simulink model "testsystem"  (R2023b)
settings: Solver=VariableStepAuto  StartTime=0.0  StopTime=50  RelTol=1e-3
values from neighbouring files (symbols this model uses):
  frontTrackWidth = 1.4    [SetVehicleParameters.m]    (also in SetVehicleParameters2.m = 1; SetVehicleParameters4.m = 1; SetVehicleParameters5.m = 1; SetVehicleParameters6.m = 1)
  g = 9.8    [SetVehicleParameters.m]    (also in SetVehicleParameters2.m; SetVehicleParameters4.m; SetVehicleParameters5.m; SetVehicleParameters6.m)
  L = Lf + Lr    (= 3)    [SetVehicleParameters.m]    (also in SetVehicleParameters2.m = 2; SetVehicleParameters4.m = 2; SetVehicleParameters5.m = 2; SetVehicleParameters6.m = 2)
  Lr = 1.6    [SetVehicleParameters.m]    (also in SetVehicleParameters2.m = 0.5; SetVehicleParameters4.m = 0.5; SetVehicleParameters5.m = 0.5; SetVehicleParameters6.m = 0.5)
  mass = 2000    [SetVehicleParameters.m]    (also in SetVehicleParameters2.m = 420; SetVehicleParameters4.m = 420; SetVehicleParameters5.m = 420; SetVehicleParameters6.m = 420)
  rearTrackWidth = 1.4    [SetVehicleParameters.m]    (also in SetVehicleParameters2.m = 1; SetVehicleParameters4.m = 1; SetVehicleParameters5.m = 1; SetVehicleParameters6.m = 1)
libraries: vehdynlibsteering x1, slpidlib x1, vehdynlibviscommon x1, SignalEditorBlockLib x1, autolibshared x1
settings Model: Creator=denoc  LastModifiedBy=denoc

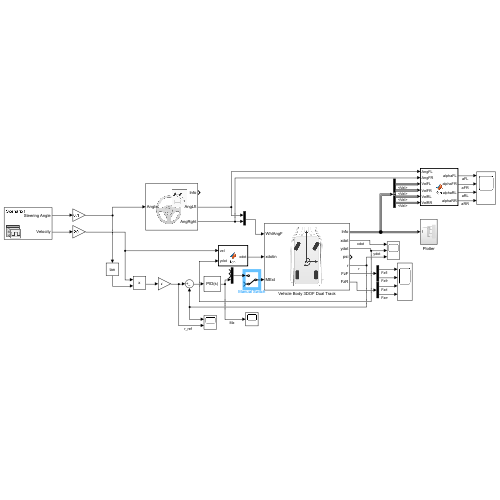
[thumbnail: Simulink's stored preview of the top-level diagram]
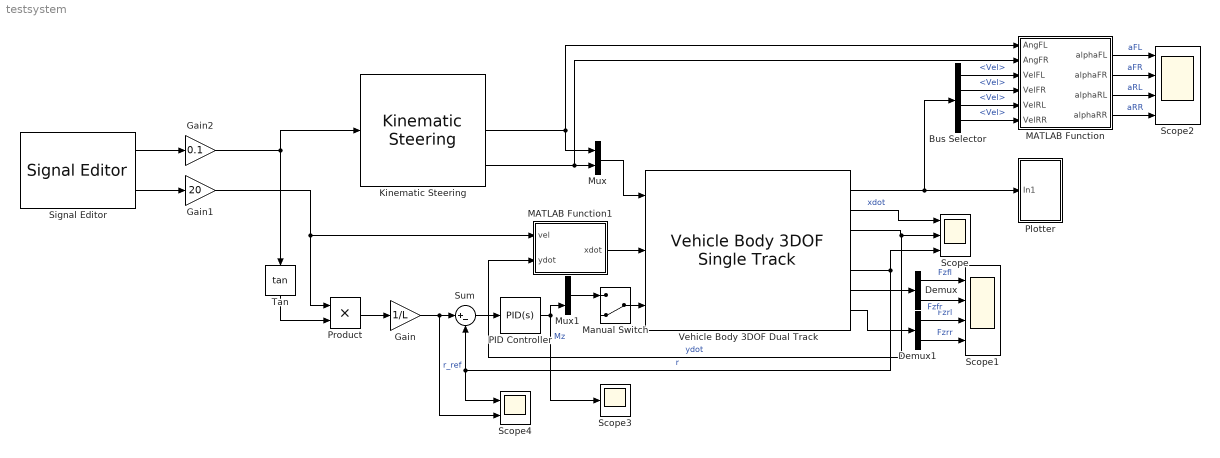
== system testsystem ==
  Bus Selector : BusSelector  OutputSignals=BdyFrm.FrntAxl.Lft.Vel,BdyFrm.FrntAxl.Rght.Vel,BdyFrm.RearAxl.Lft.Vel,BdyFrm.RearAxl.Rght.Vel
  Demux : Demux  Outputs=2
  Demux1 : Demux  Outputs=2
  Gain : Gain  Gain=1/L
  Gain1 : Gain  Gain=20
  Gain2 : Gain  Gain=0.1
  Kinematic Steering : vehdynlibsteering/Kinematic Steering  StrgType=Ackerman  StrgRatioType=Constant  Loc=Front  NrmlFctr=1  TrckWdth=frontTrackWidth  WhlBase=L  Db=0  StrgRng=1.25*pi  StrgAngBpts="[-6.2832   -5.0265   -3.7699   -2.5133   -1.2566         0    1.2566    2.5133    3.7699    5.0265    6.2832]"  StrgRatioTbl=|  StrgRatio=1  PctAckIn=off  PctAck=100  PctAckTbl=ones(1,11)*100  StrgArmLngth=0.1  RckCsLngth=0.5  TieRodLngth=0.248  D=0.2  PnnRadius=0.00085818  PnnRadiusTbl="[0.0055    0.0055    0.0056    0.0057    0.0058    0.0057    0.0057    0.0057    0.0056    0.0055    0.0055]"  RodLngth=0.1  ParaArmLngth=0.9  aMode=2
      | [13.5000   13.3750   13.2500   13.1250   13.0000   13.0000   13.0000   13.1250   13.2500   13.3750   13.5000
      | ]
  MATLAB Function : MATLAB Function  TreatAsAtomicUnit=on
  MATLAB Function1 : MATLAB Function  TreatAsAtomicUnit=on
  Manual Switch : ManualSwitch  CurrentSetting=0
  Mux : Mux  Inputs=2
  Mux1 : Mux  Inputs=3
  PID Controller : slpidlib/PID Controller  Controller=PID  Form=Parallel  TimeDomain=Continuous-time  UseExternalTs=off  SampleTime=-1  IntegratorMethod=Forward Euler  FilterMethod=Forward Euler  ControllerParametersSource=internal  P=50000  I=25000  UseKiTs=off  D=0  N=100  UseFilter=on  TunerSelectOption=Transfer Function Based (PID Tuner App)  InitialConditionSource=internal  InitialConditionForIntegrator=0  InitialConditionForFilter=0  DifferentiatorICPrevScaledInput=0  ExternalReset=none  TrackingMode=off  Kt=1  LimitOutput=off  SatLimitsSource=internal  UpperSaturationLimit=inf  LowerSaturationLimit=-inf  LinearizeAsGain=on  AntiWindupMode=none  Kb=1  LimitIntegrator=off  UpperIntegratorSaturationLimit=inf  LowerIntegratorSaturationLimit=-inf  POutMin=[]  POutMax=[]  IOutMin=[]  IOutMax=[]  DOutMin=[]  DOutMax=[]  NOutMin=[]  NOutMax=[]  SumOutMin=[]  SumOutMax=[]  SaturationOutMin=[]  SaturationOutMax=[]  PParamMin=[]  PParamMax=[]  IParamMin=[]  IParamMax=[]  DParamMin=[]  DParamMax=[]  NParamMin=[]  NParamMax=[]  KbParamMin=[]  KbParamMax=[]  KtParamMin=[]  KtParamMax=[]  KbOutMin=[]  KbOutMax=[]  KtOutMin=[]  KtOutMax=[]  IntegratorOutMin=[]  IntegratorOutMax=[]  FilterOutMin=[]  FilterOutMax=[]  SumI1OutMin=[]  SumI1OutMax=[]  SumI2OutMin=[]  SumI2OutMax=[]  SumI3OutMin=[]  SumI3OutMax=[]  SumI4OutMin=[]  SumI4OutMax=[]  SumDOutMin=[]  SumDOutMax=[]  DifferentiatorOutMin=[]  DifferentiatorOutMax=[]  FilterDiffOutCoefMin=[]  FilterDiffOutCoefMax=[]  ReciprocalOutMin=[]  ReciprocalOutMax=[]  SumDenOutMin=[]  SumDenOutMax=[]  SumNumOutMin=[]  SumNumOutMax=[]  DivideOutMin=[]  DivideOutMax=[]  UdiffTsProdOutMin=[]  UdiffTsProdOutMax=[]  NTsProdOutMin=[]  NTsProdOutMax=[]  UintegralTsProdOutMin=[]  UintegralTsProdOutMax=[]  UngainTsProdOutMin=[]  UngainTsProdOutMax=[]  ClampingZeroOutDataTypeStr=Inherit: Inherit via back propagation  ClampingZeroOutMin=[]  ClampingZeroOutMax=[]  FilterDenConstantOutDataTypeStr=Inherit: Inherit via back propagation  FilterDenConstantOutMin=[]  FilterDenConstantOutMax=[]  PCopyOutDataTypeStr=Inherit: Inherit via back propagation  PCopyOutMin=[]  PCopyOutMax=[]  NCopyOutDataTypeStr=Inherit: Inherit via back propagation  NCopyOutMin=[]  NCopyOutMax=[]  IntegratorContinuousStateAttributes=''  IntegratorStateMustResolveToSignalObject=off  IntegratorRTWStateStorageClass=Auto  FilterContinuousStateAttributes=''  FilterStateMustResolveToSignalObject=off  FilterRTWStateStorageClass=Auto  ParallelPVariant=InternalParameters  IdealPVariant=Disabled  IVariant=InternalParameters  DVariant=InternalParameters  IntegratorVariant=Continuous  SatVariant=Disabled  AWVariant=Passthrough  PCopyVariant=Disabled  TRVariant=Disabled  FdbkBlocksVariant=Forward  IdealPFdbkVariant=Disabled  SatFdbkVariant=Disabled  DerivativeFilterVariant=ContFilter  NVariant=InternalParameters  NCopyVariant=Disabled  FilterICVariant=InternalICsFilter  IntegratorICVariant=InternalICs  ExternalResetVariant=Disabled  TRSumVariant=Passthrough  SumFdbkVariant=Disabled  SumVariant=Sum_PID  TsampFilterVariant=InternalTs  TsampNgainVariant=Passthrough  TsampIntegralVariant=Disabled_SignalSpec  ExternalSaturationOutDataTypeStr=Inherit: Same as second input
  Plotter : Subsystem
  Product : Product
  Scope : Scope  NumInputPorts=3
  Scope1 : Scope  NumInputPorts=4
  Scope2 : Scope  NumInputPorts=4
  Scope3 : Scope
  Scope4 : Scope  NumInputPorts=2
  Signal Editor : SignalEditorBlockLib/Signal Editor  FileName=signals.mat  ActiveScenario=Scenario1  ActiveSignal=Steering Angle  IsBus=off  OutputBusObjectStr=Bus: BusObject  SampleTime=0  ZeroCross=off  OutputAfterFinalValue=Holding final value  Unit=inherit  PreserveSignalName=on  ApplySigPropsToAllScenarios=on  ApplySigPropsToAllSignals=on
  Sum : Sum  Inputs=|+-
  Tan : Trigonometry  Operator=tan
  Vehicle Body 3DOF Dual Track : autolibshared/Vehicle Body 3DOF Single Track  trackMode=Dual  inputMode=External longitudinal velocity  frontSteerMode=on  rearSteerMode=off  windMode=off  muMode=off  extFMode=off  extMMode=on  htchFMode=off  htchMMode=off  extXo=off  extpsio=off  extxdoto=off  extro=off  extYo=off  extTamb=off  extydoto=off  aMode=2  NF=2  NR=2  m=mass  a=Lf  b=Lr  h=h  dh=1  hh=0.2  X_o=0  xdot_o=0  CalphaMode=off  sigmaMode=on  d=0  hl=0  w=[frontTrackWidth, rearTrackWidth]  Cy_f=c_f_nom  Cy_r=c_r_nom  sigma_f=sigma_f  sigma_r=sigma_r  alpha_f_brk=[-.1 .1]  Cy_f_data=[-9e3 9e3]  alpha_r_brk=[-.1 .1]  Cy_r_data=[-9e3 9e3]  Y_o=0  ydot_o=0  Izz=Izz  psi_o=0  r_o=0  Af=2  Cd=.3  Cl=.1  Cpm=.1  beta_w=[0 0.01:0.01:0.3]  Cs=[0:0.03:0.9]  Cym=[0 1e-6:0.01:0.3]  Pabs=101325  Tair=273  g=g  mu=1  xdot_tol=.01  Fznom=Fznom  Fxtire_sat=7e4  Fytire_sat=7e4  longOff=0  latOff=0  vertOff=0  wrapAng=off
      settings: LibrarySourceBlock=vehdynlibeom/Vehicle Body 3DOF Dual Track
  wires:
  Signal Editor/1 -> Gain2/1
  Kinematic Steering/2 -> MATLAB Function/1(AngFL), Mux/1
  Kinematic Steering/3 -> MATLAB Function/2(AngFR), Mux/2
  Mux/1 -> Vehicle Body 3DOF Dual Track/1
  Vehicle Body 3DOF Dual Track/2 -> Scope/1  "xdot"
  Vehicle Body 3DOF Dual Track/3 -> MATLAB Function1/2(ydot), Scope/2  "ydot"
  Vehicle Body 3DOF Dual Track/5 -> Scope4/1, Sum/2, Scope/3  "r"
  Vehicle Body 3DOF Dual Track/1 -> Bus Selector/1, Plotter/1(In1)
  Vehicle Body 3DOF Dual Track/6 -> Demux/1
  Vehicle Body 3DOF Dual Track/7 -> Demux1/1
  Demux1/1 -> Scope1/3  "Fzrl"
  Demux1/2 -> Scope1/4  "Fzrr"
  Demux/1 -> Scope1/1  "Fzfl"
  Demux/2 -> Scope1/2  "Fzfr"
  MATLAB Function/1(alphaFL) -> Scope2/1  "aFL"
  MATLAB Function/2(alphaFR) -> Scope2/2  "aFR"
  MATLAB Function/3(alphaRL) -> Scope2/3  "aRL"
  MATLAB Function/4(alphaRR) -> Scope2/4  "aRR"
  Bus Selector/4 -> MATLAB Function/6(VelRR)  "<Vel>"
  Bus Selector/3 -> MATLAB Function/5(VelRL)  "<Vel>"
  Bus Selector/2 -> MATLAB Function/4(VelFR)  "<Vel>"
  Bus Selector/1 -> MATLAB Function/3(VelFL)  "<Vel>"
  Signal Editor/2 -> Gain1/1
  Product/1 -> Gain/1
  Gain/1 -> Scope4/2, Sum/1  "r_ref"
  Sum/1 -> PID Controller/1
  PID Controller/1 -> Scope3/1, Mux1/3  "Mz"
  Gain2/1 -> Tan/1, Kinematic Steering/1
  Gain1/1 -> MATLAB Function1/1(vel), Product/1
  MATLAB Function1/1(xdot) -> Vehicle Body 3DOF Dual Track/2
  Tan/1 -> Product/2
  Manual Switch/1 -> Vehicle Body 3DOF Dual Track/3
  Mux1/1 -> Manual Switch/1

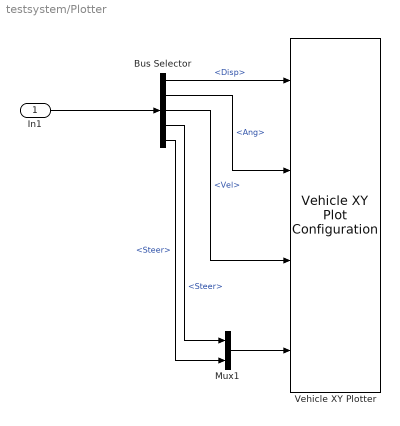
== system testsystem/Plotter ==
  In1 : Inport
  Bus Selector : BusSelector  OutputSignals=InertFrm.Cg.Disp,InertFrm.Cg.Ang,InertFrm.Cg.Vel,BdyFrm.FrntAxl.Steer,BdyFrm.RearAxl.Steer
  Mux1 : Mux  Inputs=2
  Vehicle XY Plotter : vehdynlibviscommon/Vehicle XY Plot Configuration  extRef=off  extStats=off  extTireF=off  a=Lf  b=Lr  w=rearTrackWidth  figBorder=10  bufferSize=1024  velNorm=5  tireFNorm=1000  pltDT=.1
  wires:
  Bus Selector/1 -> Vehicle XY Plotter/1  "<Disp>"
  Bus Selector/3 -> Vehicle XY Plotter/3  "<Vel>"
  Mux1/1 -> Vehicle XY Plotter/4
  Bus Selector/4 -> Mux1/1  "<Steer>"
  Bus Selector/5 -> Mux1/2  "<Steer>"
  Bus Selector/2 -> Vehicle XY Plotter/2  "<Ang>"
  In1/1 -> Bus Selector/1

== matlab function testsystem/MATLAB Function1 ==
  data: vel input; ydot input; xdot output
function xdot  = fcn(vel, ydot)

xdot = sqrt(vel^2 - ydot^2);

== matlab function testsystem/MATLAB Function ==
  data: AngFL input; AngFR input; alphaFL output; alphaFR output; alphaRL output; VelFL input; VelFR input; VelRL input; VelRR input; alphaRR output
function [alphaFL, alphaFR, alphaRL, alphaRR] = fcn(AngFL, AngFR, VelFL, VelFR, VelRL, VelRR)

alphaFL = AngFL - atan(VelFL(2) / VelFL(1));
alphaFR = AngFR - atan(VelFR(2) / VelFR(1));
alphaRL = - atan(VelRL(2) / VelRL(1));
alphaRR = - atan(VelRR(2) / VelRR(1));
